simulink model "zynqRadioHWSWQPSKAD9361AD9364SL_orig"  (R2025a)
settings: Solver=FixedStepDiscrete  StartTime=0.0  StopTime=1e6/fs  RelTol=1e-3
PreLoadFcn:
  | setTxBurstLength = 10000;
  | txtmsg = ['Zynq radio HW/SW Co-design QPSK']; % Use only printable characters
  | 
  | %------------------------------------------------------------------------------------------------------
  | if ~isequal(size(txtmsg),[1 31])
  |     error('txtmsg must contain 31 characters');
  | end
  | 
  | [dataBits,msg] = zynqRadioHWSWQPSKgenHelloworldMsg(20); % generate 20 msgs for LUT
  | msgLUT = uint8(msg);
  | dataBitsLUT = dataBits(:);
  | Rsym                = 10e3;%1.92e6;
  | Config = zynqRadioHWSWQPSKTxRxParameters;
  | fs = Rsym*Config.SamplesPerSymbol;
  | word = [txtmsg newline];  % append a new line character to txtmsg
  | 
  | % The highest clock rate is 16 times the message character rate.
  | % As the message characters are fed at highest clock to FPGA
  | % repeat each character 16 times to maintain the message rate.
  | word = repelem(word.',16,1);
  | repeatTimes = ceil(setTxBurstLength/length(word));
  | inpData = complex(repmat(uint8(word),repeatTimes,1));
  | inUseTxBurstLength = length(inpData);
PostLoadFcn:
  | hScopeConfig = get_param([gcs '/HDL_QPSK/QPSK Tx Channel QPSK Rx/QPSK Rx/Frequency and Time Synchronizer/Symbol Synchronizer/No HDL/QPSK Receiver Eye Diagram'],'ScopeConfiguration');
  | hScopeConfig.OpenAtSimulationStart = false;
  | hScopeConfig.Visible = false;
  | clear hScopeConfig
InitFcn:
  | setTxBurstLength = 10000;
  | txtmsg = ['Zynq radio HW/SW Co-design QPSK']; % Use only printable characters
  | 
  | %------------------------------------------------------------------------------------------------------
  | if ~isequal(size(txtmsg),[1 31])
  |     error('txtmsg must contain 31 characters');
  | end
  | 
  | [dataBits,msg] = zynqRadioHWSWQPSKgenHelloworldMsg(20); % generate 20 msgs for LUT
  | msgLUT = uint8(msg);
  | dataBitsLUT = dataBits(:);
  | Rsym                = 10e3;%1.92e6;
  | Config = zynqRadioHWSWQPSKTxRxParameters;
  | fs = Rsym*Config.SamplesPerSymbol;
  | word = [txtmsg newline];  % append a new line character to txtmsg
  | 
  | % The highest clock rate is 16 times the message character rate.
  | % As the message characters are fed at highest clock to FPGA
  | % repeat each character 16 times to maintain the message rate.
  | word = repelem(word.',16,1);
  | repeatTimes = ceil(setTxBurstLength/length(word));
  | inpData = complex(repmat(uint8(word),repeatTimes,1));
  | inUseTxBurstLength = length(inpData);
undefined symbols (not defined in the file or in its folder): Add, DSP48_Variant, dspblkCoreblockFVToolHelper, gcbh, NCO_DUT, Shift, xc7z020clg484
libraries: hdlsllib x84, hdlBasic x50, simulink x34, dsphdlsigops2 x3, dsphdlfiltering2 x3, dsphdlxfrm2 x2, dsphdlmathfun2 x2, commdigbbndpm3 x2, vmcUtilities x1, sdrzblksprivate x1
(part 1 of 4)
CloseFcn:
  | clear Config dataBits dataBitsLUT fs h inpData ...
  |         inUseTxBurstLength msg msgLUT repeatTimes ...
  |         Rsym setTxBurstLength simAfterCS simBeforeSS ...
  |         simPeakFind simSyncedPackets simTimingOffset ...
  |         simUserData tout txtmsg word captureASCII
settings Model: DataTypeOverride=Off  Creator=The MathWorks, Inc.  LastModifiedBy=daniel
settings DataIOCC: ReturnWorkspaceOutputs=off
settings OptimizationCC: BlockReduction=off  ConditionallyExecuteInputs=off  DefaultParameterBehavior=Inlined  InheritOutputTypeSmallerThanSingle=on  ReuseModelBlockBuffer=off
settings DebuggingCC: AlgebraicLoopMsg=error  SingleTaskRateTransMsg=error  SubsystemReferenceDiagnosticForUnitTest=warning
settings HardwareCC: ProdBitPerPointer=32.0  ProdBitPerSizeT=32.0  ProdBitPerPtrDiffT=32.0  ProdLargestAtomicFloat=None  ProdIntDivRoundTo=Undefined  ProdEndianess=Unspecified  ProdWordSize=32.0  ProdHWDeviceType=ASIC/FPGA->ASIC/FPGA  TargetBitPerLong=64.0  TargetBitPerPointer=64.0  TargetBitPerSizeT=64.0  TargetBitPerPtrDiffT=64.0  TargetLongLongMode=on  TargetIntDivRoundTo=Zero  TargetEndianess=LittleEndian  TargetWordSize=64.0  TargetHWDeviceType=Custom Processor->MATLAB Host Computer  ProdEqTarget=off
settings RTWCC: GPUComputeCapability=3.5

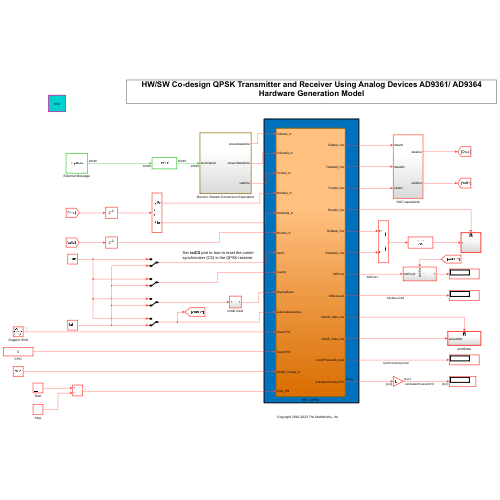
[thumbnail: Simulink's stored preview of the top-level diagram]
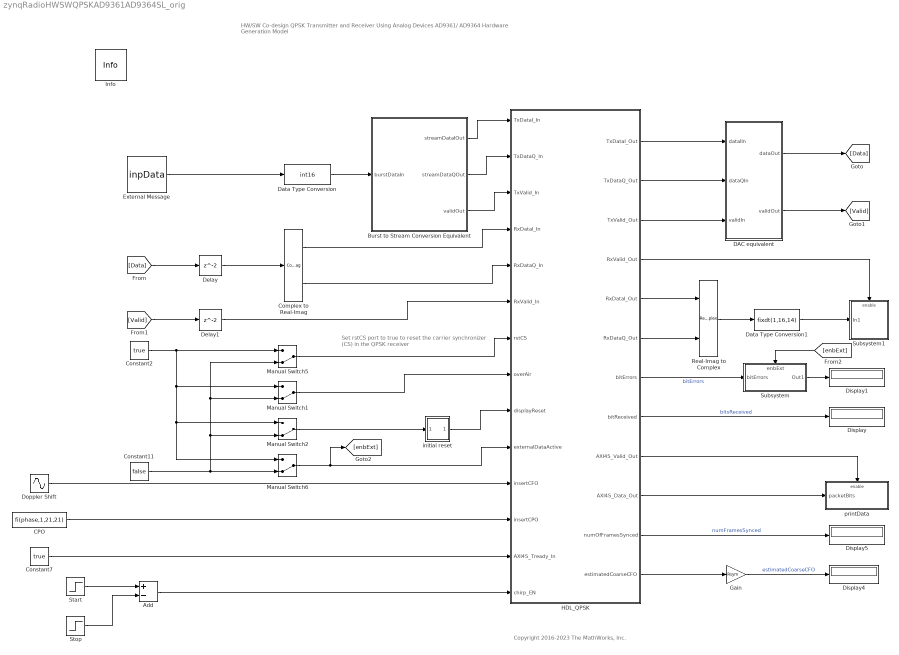
== system zynqRadioHWSWQPSKAD9361AD9364SL_orig ==
  note: Set rstCS port to true to reset the carrier synchronizer (CS) in the QPSK receiver
  note: Copyright 2016-2023 The MathWorks, Inc.
  note: HW/SW Co-design QPSK Transmitter and Receiver Using Analog Devices AD9361/ AD9364
      | Hardware Generation Model
  Add : Sum  Inputs=+-
  Burst to Stream Conversion Equivalent : Subsystem
  CPO : Constant  Value=fi(phase,1,21,21)  SampleTime=1/fs  mask{phased=0}
      mask prompts: phased "CPO (degrees):"
      mask init:
      | phase = phased/360;
      mask DialogControl DescGroupVar Prompt: Insert CPO
      mask DialogControl DescTextVar Prompt: Introduce CPO into transmitter waveform. The overAir port must be set to false. CPO range: -180 to less than 180
      mask Display: disp(get_param(gcb,"phased"));
  Complex to Real-Imag : ComplexToRealImag
  Constant11 : Constant  Value=false  OutDataTypeStr=boolean  SampleTime=1/fs
  Constant2 : Constant  Value=true  OutDataTypeStr=boolean  SampleTime=1/fs
  Constant7 : Constant  Value=true  OutDataTypeStr=boolean  SampleTime=1/fs
  DAC equivalent : Subsystem
  Data Type Conversion : DataTypeConversion  OutDataTypeStr=int16  SaturateOnIntegerOverflow=off  RndMeth=Floor
  Data Type Conversion1 : DataTypeConversion  OutDataTypeStr=fixdt(1,16,14)  ConvertRealWorld=Stored Integer (SI)  SaturateOnIntegerOverflow=off  RndMeth=Floor
  Delay : Delay
  Delay1 : Delay
  Display{,1,4..5} (4 alike) : Display
  Doppler Shift : Sin  SineType=Sample based  Amplitude=-100e3  Bias=100e3  Frequency=2*pi  Phase=pi  Samples=5*60*fs  SampleTime=1/fs
  External Message : Constant  Value=inpData  SampleTime=-1
  Gain : Gain  Gain=Rsym  OutDataTypeStr=double
  HDL_QPSK : Subsystem  TreatAsAtomicUnit=on
  Info : sdrzblksprivate/Info  SystemSampleTime=-1  VariantActivationTime=update diagram  EmptyChoice=off  PassThrough=off  PassThroughVariantControl=(default)  EmptyChoiceVariantControl=(default)  AllowFlexibleInterface=on  Latency=0  AutoFrameSizeCalculation=off
  Manual Switch{1..2,5..6} (4 alike) : ManualSwitch  CurrentSetting=0
  Real-Imag to Complex : RealImagToComplex
  Start : Step  Time=200e3/fs  SampleTime=1/fs
  Stop : Step  Time=400e3/fs  SampleTime=1/fs
  Subsystem : Subsystem
      settings: PortSchema="{\"entries\":[{\"content\":{\"sides\":[{\"content\":{\"connectorIds\":[\"In1\"]},\"type\":\"ConnectorPlacement.EquallySpacedRectSide\",\"uuid\":\"00e2ba4b-7eac-479c-adca-0b3a47f26300\"},{\"content\":{\"connectorIds\":[\"Out1\"],\"side\":\"RIGHT\"},\"type\":\"ConnectorPlacement.EquallySpacedRectSide\",\"uuid\":\"f46d1850-7aaf-4a4a-a0f0-18f53e4dd1ab\"},{\"content\":{\"connectorIds\":[\"In2\"],\"side\":\"TOP\"},\"type\":\"ConnectorPlacement.EquallySpacedRectSide\",\"uuid\":\"6eb79df9-d0ed-4616-8b56-bf03dd754f89\"}]},\"type\":\"ConnectorPlacement.EquallySpacedConnector\",\"uuid\":\"71623fc3-6fb3-42f9-b5c9-cd74da1aa0dd\"}],\"packageUris\":[\"http://schema.mathworks.com/mf0/Connector/R2020b\"],\"version\":\"1.0\"}"
  Subsystem1 : Subsystem
  initial reset : Subsystem
  printData : Subsystem
  wires:
  Doppler Shift/1 -> HDL_QPSK/11(insertCFO)
  Subsystem/1(Out1) -> Display1/1
  Complex to Real-Imag/1 -> HDL_QPSK/4(RxDataI_In)
  HDL_QPSK/1(TxDataI_Out) -> DAC equivalent/1(dataIIn)
  DAC equivalent/1(dataOut) -> [Data]
  [Valid] -> Delay1/1
  HDL_QPSK/2(TxDataQ_Out) -> DAC equivalent/2(dataQIn)
  HDL_QPSK/6(RxDataQ_Out) -> Real-Imag to Complex/2
  Manual Switch5/1 -> HDL_QPSK/7(rstCS)
  HDL_QPSK/12(estimatedCoarseCFO) -> Gain/1
  Delay1/1 -> HDL_QPSK/6(RxValid_In)
  CPO/1 -> HDL_QPSK/12(insertCPO)
  Manual Switch1/1 -> HDL_QPSK/8(overAir)
  HDL_QPSK/9(AXI4S_Valid_Out) -> printData/Enable
  Real-Imag to Complex/1 -> Data Type Conversion1/1
  Data Type Conversion1/1 -> Subsystem1/1(In1)
  HDL_QPSK/4(RxValid_Out) -> Subsystem1/Enable
  HDL_QPSK/10(AXI4S_Data_Out) -> printData/1(packetBits)
  External Message/1 -> Data Type Conversion/1
  Constant7/1 -> HDL_QPSK/13(AXI4S_Tready_In)
  Burst to Stream Conversion Equivalent/3(validOut) -> HDL_QPSK/3(TxValid_In)
  DAC equivalent/2(validOut) -> [Valid]
  Burst to Stream Conversion Equivalent/1(streamDataIOut) -> HDL_QPSK/1(TxDataI_In)
  Gain/1 -> Display4/1  "estimatedCoarseCFO"
  Delay/1 -> Complex to Real-Imag/1
  HDL_QPSK/7(bitErrors) -> Subsystem/1(bitErrors)  "bitErrors"
  HDL_QPSK/11(numOfFramesSynced) -> Display5/1  "numFramesSynced"
  HDL_QPSK/3(TxValid_Out) -> DAC equivalent/3(validIn)
  [enbExt] -> Subsystem/2(enbExt)
  Manual Switch2/1 -> initial reset/1(In2)
  initial reset/1(Out1) -> HDL_QPSK/9(displayReset)
  Constant2/1 -> Manual Switch6/1, Manual Switch2/1, Manual Switch1/1, Manual Switch5/1
  Burst to Stream Conversion Equivalent/2(streamDataQOut) -> HDL_QPSK/2(TxDataQ_In)
  Constant11/1 -> Manual Switch6/2, Manual Switch5/2, Manual Switch1/2, Manual Switch2/2
  HDL_QPSK/5(RxDataI_Out) -> Real-Imag to Complex/1
  Data Type Conversion/1 -> Burst to Stream Conversion Equivalent/1(burstDataIn)
  Complex to Real-Imag/2 -> HDL_QPSK/5(RxDataQ_In)
  HDL_QPSK/8(bitReceived) -> Display/1  "bitsReceived"
  [Data] -> Delay/1
  Manual Switch6/1 -> HDL_QPSK/10(externalDataActive), [enbExt]
  Start/1 -> Add/1
  Stop/1 -> Add/2
  Add/1 -> HDL_QPSK/14(chirp_EN)

== system zynqRadioHWSWQPSKAD9361AD9364SL_orig/Burst to Stream Conversion Equivalent ==
  note: The burst data sent from the processing system will be stored in the RAM in the memory channel of SDR IIO radio. The data stored will be poped out as a stream data.
  note: This subsystem does an equivalent operation to simulate the input and output behaviour of the memory channel of the SDR IIO radio.
  burstDataIn : Inport
  Complex to Real-Imag : ComplexToRealImag
  Serializer1D : hdlsllib/HDL Operations/Serializer1D  Ratio=inUseTxBurstLength  IdleCycles=0  validIn=off  startOut=off  validOut=on  inputDataDimensions=-1  inputSampleTime=-1  inputSignalType=auto
  streamDataIOut : Outport
  streamDataQOut : Outport  Port=2
  validOut : Outport  Port=3
  wires:
  burstDataIn/1 -> Serializer1D/1
  Serializer1D/1 -> Complex to Real-Imag/1
  Complex to Real-Imag/1 -> streamDataIOut/1
  Complex to Real-Imag/2 -> streamDataQOut/1
  Serializer1D/2 -> validOut/1

== system zynqRadioHWSWQPSKAD9361AD9364SL_orig/DAC equivalent ==
  dataIIn : Inport
  dataQIn : Inport  Port=2
  validIn : Inport  Port=3
  Data Type Conversion : DataTypeConversion  OutDataTypeStr=int16  SaturateOnIntegerOverflow=off  RndMeth=Floor
  Extract Bits : simulink/Logic and Bit Operations/Extract Bits  bitsToExtract=Range starting with most significant bit  numBits=12  bitIdxRange=[0 7]  outScalingMode=Treat bit field as an integer
  Extract Bits1 : simulink/Logic and Bit Operations/Extract Bits  bitsToExtract=Range starting with most significant bit  numBits=12  bitIdxRange=[0 7]  outScalingMode=Treat bit field as an integer
  Real-Imag to Complex : RealImagToComplex
  dataOut : Outport
  validOut : Outport  Port=2
  wires:
  dataIIn/1 -> Extract Bits/1
  dataQIn/1 -> Extract Bits1/1
  Extract Bits/1 -> Real-Imag to Complex/1
  Extract Bits1/1 -> Real-Imag to Complex/2
  Real-Imag to Complex/1 -> Data Type Conversion/1
  validIn/1 -> validOut/1
  Data Type Conversion/1 -> dataOut/1

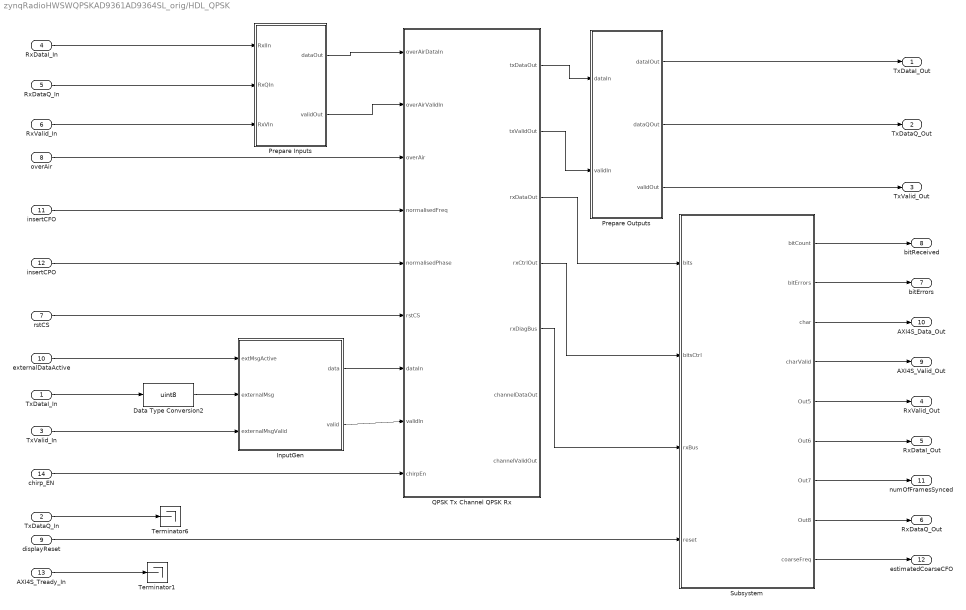
== system zynqRadioHWSWQPSKAD9361AD9364SL_orig/HDL_QPSK ==
  TxDataI_In : Inport
  TxDataQ_In : Inport  Port=2
  TxValid_In : Inport  Port=3
  RxDataI_In : Inport  Port=4
  RxDataQ_In : Inport  Port=5
  RxValid_In : Inport  Port=6
  rstCS : Inport  Port=7
  overAir : Inport  Port=8
  displayReset : Inport  Port=9
  externalDataActive : Inport  Port=10
  insertCFO : Inport  Port=11
  insertCPO : Inport  Port=12
  AXI4S_Tready_In : Inport  Port=13
  chirp_EN : Inport  Port=14
  Data Type Conversion2 : DataTypeConversion  OutDataTypeStr=uint8  SaturateOnIntegerOverflow=off  RndMeth=Floor
  InputGen : Subsystem
  Prepare Inputs : Subsystem
  Prepare Outputs : Subsystem
  QPSK Tx Channel QPSK Rx : Subsystem
  Subsystem : Subsystem
  Terminator1 : Terminator
  Terminator6 : Terminator
  TxDataI_Out : Outport
  TxDataQ_Out : Outport  Port=2
  TxValid_Out : Outport  Port=3
  RxValid_Out : Outport  Port=4
  RxDataI_Out : Outport  Port=5
  RxDataQ_Out : Outport  Port=6
  bitErrors : Outport  Port=7
  bitReceived : Outport  Port=8
  AXI4S_Valid_Out : Outport  Port=9
  AXI4S_Data_Out : Outport  Port=10
  numOfFramesSynced : Outport  Port=11
  estimatedCoarseCFO : Outport  Port=12
  wires:
  Prepare Outputs/2(dataQOut) -> TxDataQ_Out/1
  Prepare Outputs/3(validOut) -> TxValid_Out/1
  AXI4S_Tready_In/1 -> Terminator1/1
  Prepare Inputs/1(dataOut) -> QPSK Tx Channel QPSK Rx/1(overAirDataIn)
  Prepare Inputs/2(validOut) -> QPSK Tx Channel QPSK Rx/2(overAirValidIn)
  InputGen/1(data) -> QPSK Tx Channel QPSK Rx/7(dataIn)
  InputGen/2(valid) -> QPSK Tx Channel QPSK Rx/8(validIn)
  overAir/1 -> QPSK Tx Channel QPSK Rx/3(overAir)
  insertCFO/1 -> QPSK Tx Channel QPSK Rx/4(normalisedFreq)
  insertCPO/1 -> QPSK Tx Channel QPSK Rx/5(normalisedPhase)
  QPSK Tx Channel QPSK Rx/1(txDataOut) -> Prepare Outputs/1(dataIn)
  QPSK Tx Channel QPSK Rx/2(txValidOut) -> Prepare Outputs/2(validIn)
  displayReset/1 -> Subsystem/4(reset)
  QPSK Tx Channel QPSK Rx/3(rxDataOut) -> Subsystem/1(bits)
  QPSK Tx Channel QPSK Rx/4(rxCtrlOut) -> Subsystem/2(bitsCtrl)
  QPSK Tx Channel QPSK Rx/5(rxDiagBus) -> Subsystem/3(rxBus)
  Subsystem/1(bitCount) -> bitReceived/1
  Subsystem/2(bitErrors) -> bitErrors/1
  Subsystem/3(char) -> AXI4S_Data_Out/1
  Subsystem/4(charValid) -> AXI4S_Valid_Out/1
  Subsystem/5(Out5) -> RxValid_Out/1
  Subsystem/6(Out6) -> RxDataI_Out/1
  Subsystem/7(Out7) -> numOfFramesSynced/1
  Subsystem/8(Out8) -> RxDataQ_Out/1
  rstCS/1 -> QPSK Tx Channel QPSK Rx/6(rstCS)
  Subsystem/9(coarseFreq) -> estimatedCoarseCFO/1
  Prepare Outputs/1(dataIOut) -> TxDataI_Out/1
  RxDataI_In/1 -> Prepare Inputs/1(RxIIn)
  RxDataQ_In/1 -> Prepare Inputs/2(RxQIn)
  RxValid_In/1 -> Prepare Inputs/3(RxVIn)
  TxValid_In/1 -> InputGen/3(externalMsgValid)
  TxDataQ_In/1 -> Terminator6/1
  externalDataActive/1 -> InputGen/1(extMsgActive)
  TxDataI_In/1 -> Data Type Conversion2/1
  Data Type Conversion2/1 -> InputGen/2(externalMsg)
  chirp_EN/1 -> QPSK Tx Channel QPSK Rx/9(chirpEn)

== system zynqRadioHWSWQPSKAD9361AD9364SL_orig/Subsystem ==
  note: 2^32-1 will be treated as NaN in double when converted to double
  bitErrors : Inport
  enbExt : Inport  Port=2
  Compare To Constant : simulink/Logic and Bit Operations/Compare To Constant  relop===  const=2^32-1  OutDataTypeStr=boolean
  Constant : Constant  Value=2^32-1  OutDataTypeStr=uint32  SampleTime=-1
  Constant1 : Constant  Value=NaN  SampleTime=-1
  Data Type Conversion3 : DataTypeConversion  OutDataTypeStr=double  SaturateOnIntegerOverflow=off  RndMeth=Floor
  Switch : Switch  Criteria=u2 ~= 0  SaturateOnIntegerOverflow=off  InputSameDT=off
  Switch1 : Switch  Criteria=u2 ~= 0  SaturateOnIntegerOverflow=off  InputSameDT=off
  Out1 : Outport
  wires:
  Constant/1 -> Switch/1
  bitErrors/1 -> Switch/3
  enbExt/1 -> Switch/2
  Compare To Constant/1 -> Switch1/2
  Switch1/1 -> Out1/1
  Switch/1 -> Data Type Conversion3/1, Compare To Constant/1
  Data Type Conversion3/1 -> Switch1/3
  Constant1/1 -> Switch1/1

== system zynqRadioHWSWQPSKAD9361AD9364SL_orig/Subsystem1 ==
  In1 : Inport
  Enable : EnablePort
  Constellation Diagram : ConstellationDiagram  WindowPosition=[499.000000,206.000000,1692.000000,1017.000000,]  ScopeFrameLocation=window  SymbolsToDisplaySource=Property  SymbolsToDisplay=10000  XLimits=[-1.38,1.38]  YLimits=[-1.38,1.38]  AxesLimits=[-1.38,1.38]  DefaultConfigurationName=comm.scopes.ConstellationDiagramBlockCfg
  Terminator : Terminator
  wires:
  In1/1 -> Constellation Diagram/1, Terminator/1

== system zynqRadioHWSWQPSKAD9361AD9364SL_orig/initial reset ==
  In2 : Inport
  Constant : Constant  OutDataTypeStr=boolean  SampleTime=-1
  Delay : Delay  DelayLength=1
  Logical Operator : Logic  Operator=OR  IconShape=distinctive  AllPortsSameDT=off  OutDataTypeStr=boolean
  Logical Operator1 : Logic  Operator=XOR  IconShape=distinctive  AllPortsSameDT=off  OutDataTypeStr=boolean
  Out1 : Outport
  wires:
  In2/1 -> Logical Operator/2
  Logical Operator1/1 -> Logical Operator/1
  Logical Operator/1 -> Out1/1
  Constant/1 -> Delay/1, Logical Operator1/1
  Delay/1 -> Logical Operator1/2

== system zynqRadioHWSWQPSKAD9361AD9364SL_orig/printData ==
  packetBits : Inport
  Enable : EnablePort
  Extract Bits : simulink/Logic and Bit Operations/Extract Bits  bitsToExtract=Range ending with least significant bit  numBits=8  bitIdxRange=[0 7]  outScalingMode=Treat bit field as an integer
  MATLAB Function : MATLAB Function  TreatAsAtomicUnit=on
  Serializer1D : hdlsllib/HDL Operations/Serializer1D  Ratio=1  IdleCycles=0  validIn=off  startOut=off  validOut=off  inputDataDimensions=-1  inputSampleTime=-1  inputSignalType=auto
  captureASCII : ToWorkspace  VariableName=captureASCII  SampleTime=-1
      settings: Save2DSignal=2-D array (concatenate along first dimension)
  wires:
  packetBits/1 -> Serializer1D/1
  Serializer1D/1 -> Extract Bits/1
  Extract Bits/1 -> captureASCII/1, MATLAB Function/1(u)

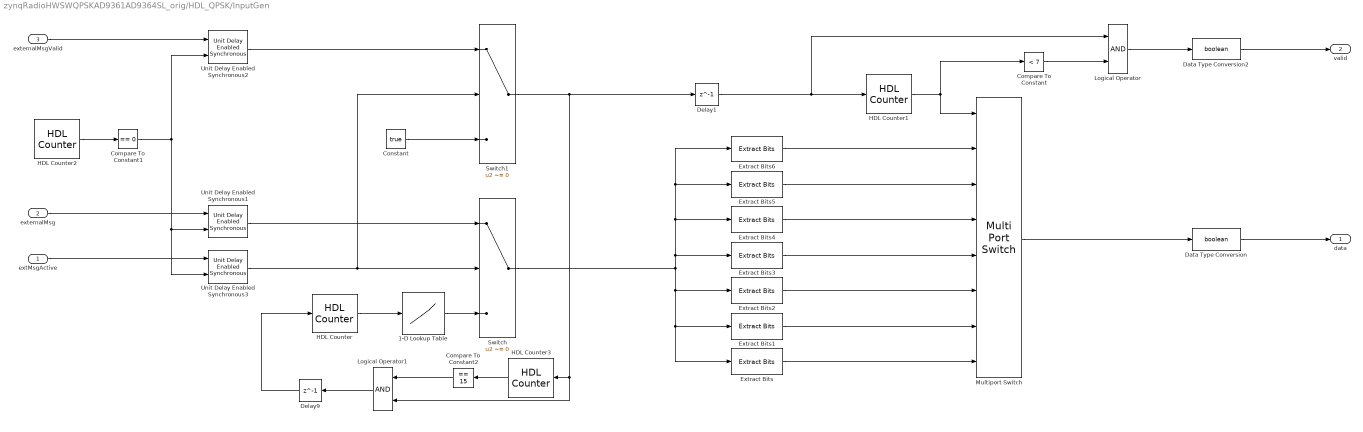
== system zynqRadioHWSWQPSKAD9361AD9364SL_orig/HDL_QPSK/InputGen ==
  extMsgActive : Inport
  externalMsg : Inport  Port=2
  externalMsgValid : Inport  Port=3
  1-D Lookup Table : Lookup_n-D  NumberOfTableDimensions=1  LookupTableObject=''  BreakpointsForDimension1=0:length(msgLUT) - 1  BreakpointsForDimension1FirstPoint=10  BreakpointsForDimension2FirstPoint=10  BreakpointsForDimension1Spacing=12  BreakpointsForDimension2Spacing=12  IndexSearchMethod=Evenly spaced points  Table=msgLUT  TableDataTypeStr=uint8  InterpMethod=Flat  DiagnosticForOutOfRangeInput=Error  InternalRulePriority=Speed  OutDataTypeStr=uint8  RndMeth=Simplest
  Compare To Constant : simulink/Logic and Bit Operations/Compare To Constant  relop=<  const=7  OutDataTypeStr=boolean
  Compare To Constant1 : hdlsllib/Logic and Bit Operations/Compare To Constant  relop===  const=0  OutDataTypeStr=boolean
  Compare To Constant2 : hdlsllib/Logic and Bit Operations/Compare To Constant  relop===  const=15  OutDataTypeStr=boolean
  Constant : Constant  Value=true  SampleTime=-1
  Data Type Conversion : DataTypeConversion  OutDataTypeStr=boolean  SaturateOnIntegerOverflow=off  RndMeth=Floor
  Data Type Conversion2 : DataTypeConversion  OutDataTypeStr=boolean  SaturateOnIntegerOverflow=off  RndMeth=Floor
  Delay1 : Delay  DelayLength=1
  Delay9 : Delay  DelayLength=1
  Extract Bits : simulink/Logic and Bit Operations/Extract Bits  bitsToExtract=Range of bits  numBits=8  bitIdxRange=0  outScalingMode=Treat bit field as an integer
  Extract Bits1 : simulink/Logic and Bit Operations/Extract Bits  bitsToExtract=Range of bits  numBits=8  bitIdxRange=1  outScalingMode=Treat bit field as an integer
  Extract Bits2 : simulink/Logic and Bit Operations/Extract Bits  bitsToExtract=Range of bits  numBits=8  bitIdxRange=2  outScalingMode=Treat bit field as an integer
  Extract Bits3 : simulink/Logic and Bit Operations/Extract Bits  bitsToExtract=Range of bits  numBits=8  bitIdxRange=3  outScalingMode=Treat bit field as an integer
  Extract Bits4 : simulink/Logic and Bit Operations/Extract Bits  bitsToExtract=Range of bits  numBits=8  bitIdxRange=4  outScalingMode=Treat bit field as an integer
  Extract Bits5 : simulink/Logic and Bit Operations/Extract Bits  bitsToExtract=Range of bits  numBits=8  bitIdxRange=5  outScalingMode=Treat bit field as an integer
  Extract Bits6 : simulink/Logic and Bit Operations/Extract Bits  bitsToExtract=Range of bits  numBits=8  bitIdxRange=6  outScalingMode=Treat bit field as an integer
  HDL Counter : hdlsllib/Sources/HDL Counter  CountType=Count limited  CountInit=0  CountStep=1  CountMax=length(msgLUT) - 1  CountFromType=Initial value  CountFrom=0  CountResetPort=off  CountLoadPort=off  CountEnbPort=on  CountDirPort=off  CountHitOutputPort=off  CountDataType=Unsigned  CountWordLen=nextpow2(length(msgLUT) - 1)  CountFracLen=0  CountSampTime=8/(Rsym*2)
  HDL Counter1 : hdlsllib/Sources/HDL Counter  CountType=Count limited  CountInit=0  CountStep=1  CountMax=15  CountFromType=Initial value  CountFrom=0  CountResetPort=off  CountLoadPort=off  CountEnbPort=on  CountDirPort=off  CountHitOutputPort=off  CountDataType=Unsigned  CountWordLen=4  CountFracLen=0  CountSampTime=1
  HDL Counter2 : hdlsllib/Sources/HDL Counter  CountType=Count limited  CountInit=0  CountStep=1  CountMax=15  CountFromType=Initial value  CountFrom=0  CountResetPort=off  CountLoadPort=off  CountEnbPort=off  CountDirPort=off  CountHitOutputPort=off  CountDataType=Unsigned  CountWordLen=4  CountFracLen=0  CountSampTime=1/fs
  HDL Counter3 : hdlsllib/Sources/HDL Counter  CountType=Count limited  CountInit=0  CountStep=1  CountMax=15  CountFromType=Initial value  CountFrom=0  CountResetPort=off  CountLoadPort=off  CountEnbPort=on  CountDirPort=off  CountHitOutputPort=off  CountDataType=Unsigned  CountWordLen=4  CountFracLen=0  CountSampTime=1/fs
  Logical Operator : Logic  AllPortsSameDT=off  OutDataTypeStr=boolean
  Logical Operator1 : Logic  AllPortsSameDT=off  OutDataTypeStr=boolean
  Multiport Switch : MultiPortSwitch  DataPortOrder=Zero-based contiguous  Inputs=7  DiagnosticForDefault=None  zeroidx=on  SaturateOnIntegerOverflow=off  InputSameDT=off
  Switch : Switch  Criteria=u2 ~= 0  SaturateOnIntegerOverflow=off  InputSameDT=off
  Switch1 : Switch  Criteria=u2 ~= 0  SaturateOnIntegerOverflow=off  InputSameDT=off
  Unit Delay Enabled Synchronous1 : hdlsllib/Discrete/Unit Delay Enabled Synchronous  InitialCondition=0.0  SampleTime=-1
  Unit Delay Enabled Synchronous2 : hdlsllib/Discrete/Unit Delay Enabled Synchronous  InitialCondition=0.0  SampleTime=-1
  Unit Delay Enabled Synchronous3 : hdlsllib/Discrete/Unit Delay Enabled Synchronous  InitialCondition=0.0  SampleTime=-1
  data : Outport
  valid : Outport  Port=2
  wires:
  Logical Operator1/1 -> Delay9/1
  Compare To Constant2/1 -> Logical Operator1/1
  HDL Counter3/1 -> Compare To Constant2/1
  Delay1/1 -> Logical Operator/1, HDL Counter1/1
  Constant/1 -> Switch1/3
  Extract Bits/1 -> Multiport Switch/8
  Extract Bits1/1 -> Multiport Switch/7
  Extract Bits2/1 -> Multiport Switch/6
  Extract Bits3/1 -> Multiport Switch/5
  Extract Bits4/1 -> Multiport Switch/4
  Extract Bits5/1 -> Multiport Switch/3
  Extract Bits6/1 -> Multiport Switch/2
  Unit Delay Enabled Synchronous3/1 -> Switch/2, Switch1/2
  extMsgActive/1 -> Unit Delay Enabled Synchronous3/1
  Unit Delay Enabled Synchronous2/1 -> Switch1/1
  externalMsg/1 -> Unit Delay Enabled Synchronous1/1
  Compare To Constant1/1 -> Unit Delay Enabled Synchronous1/2, Unit Delay Enabled Synchronous3/2, Unit Delay Enabled Synchronous2/2
  externalMsgValid/1 -> Unit Delay Enabled Synchronous2/1
  HDL Counter2/1 -> Compare To Constant1/1
  Unit Delay Enabled Synchronous1/1 -> Switch/1
  Delay9/1 -> HDL Counter/1
  Switch/1 -> Extract Bits3/1, Extract Bits4/1, Extract Bits5/1, Extract Bits6/1, Extract Bits2/1, Extract Bits1/1, Extract Bits/1
  Logical Operator/1 -> Data Type Conversion2/1
  Switch1/1 -> Delay1/1, HDL Counter3/1, Logical Operator1/2
  1-D Lookup Table/1 -> Switch/3
  Compare To Constant/1 -> Logical Operator/2
  HDL Counter1/1 -> Multiport Switch/1, Compare To Constant/1
  Multiport Switch/1 -> Data Type Conversion/1
  HDL Counter/1 -> 1-D Lookup Table/1
  Data Type Conversion/1 -> data/1
  Data Type Conversion2/1 -> valid/1

== system zynqRadioHWSWQPSKAD9361AD9364SL_orig/HDL_QPSK/Prepare Inputs ==
  RxIIn : Inport
  RxQIn : Inport  Port=2
  RxVIn : Inport  Port=3
  Data Type Conversion5 : DataTypeConversion  OutDataTypeStr=fixdt(1,16,14)  ConvertRealWorld=Stored Integer (SI)  SaturateOnIntegerOverflow=off  RndMeth=Floor
  Delay{1,3..4,6} (4 alike) : Delay
  Delay2 : Delay  DelayLength=4
  Delay5 : Delay  DelayLength=4
  Gain : Gain  Gain=16  ParamDataTypeStr=fixdt(0,5,0)  OutDataTypeStr=Inherit: Same as input
  Real-Imag to Complex : RealImagToComplex
  dataOut : Outport
  validOut : Outport  Port=2
  wires:
  RxIIn/1 -> Real-Imag to Complex/1
  Gain/1 -> Delay2/1
  Real-Imag to Complex/1 -> Data Type Conversion5/1
  Delay5/1 -> Delay6/1
  Data Type Conversion5/1 -> Delay1/1
  Delay2/1 -> Delay3/1
  Delay4/1 -> Delay5/1
  RxQIn/1 -> Real-Imag to Complex/2
  Delay1/1 -> Gain/1
  RxVIn/1 -> Delay4/1
  Delay6/1 -> validOut/1
  Delay3/1 -> dataOut/1

== system zynqRadioHWSWQPSKAD9361AD9364SL_orig/HDL_QPSK/Prepare Outputs ==
  dataIn : Inport
  validIn : Inport  Port=2
  Complex to Real-Imag1 : ComplexToRealImag
  Data Type Conversion4 : DataTypeConversion  OutDataTypeStr=int16  ConvertRealWorld=Stored Integer (SI)  SaturateOnIntegerOverflow=off  RndMeth=Floor
  Delay7 : Delay
  Delay8 : Delay
  Delay9 : Delay
  dataIOut : Outport
  dataQOut : Outport  Port=2
  validOut : Outport  Port=3
  wires:
  dataIn/1 -> Data Type Conversion4/1
  Delay7/1 -> dataIOut/1
  Complex to Real-Imag1/2 -> Delay8/1
  validIn/1 -> Delay9/1
  Complex to Real-Imag1/1 -> Delay7/1
  Data Type Conversion4/1 -> Complex to Real-Imag1/1
  Delay9/1 -> validOut/1
  Delay8/1 -> dataQOut/1

== system zynqRadioHWSWQPSKAD9361AD9364SL_orig/HDL_QPSK/QPSK Tx Channel QPSK Rx ==
  overAirDataIn : Inport
  overAirValidIn : Inport  Port=2
  overAir : Inport  Port=3
  normalisedFreq : Inport  Port=4
  normalisedPhase : Inport  Port=5
  rstCS : Inport  Port=6
  dataIn : Inport  Port=7
  validIn : Inport  Port=8
  chirpEn : Inport  Port=9
  Data Type Conversion7 : DataTypeConversion  OutDataTypeStr=fixdt(1,16,14)  SaturateOnIntegerOverflow=off  RndMeth=Floor
  QPSK Rx : Subsystem
      mask init:
      | integAvgLen = 2^15;
      | 
      | RxParams            = zynqRadioHWSWQPSKTxRxParameters();
      | Preamble            = RxParams.Preamble;
      | QPSKConstellation   = RxParams.QPSKConstellation;
      | dataBitsPerPacket   = RxParams.DataBitsPerPacket;
      | SamplesPerSymbol    = RxParams.SamplesPerSymbol;
      | RRCCoef             = RxParams.RRCCoef;
      | bitsPerPacket        = RxParams.BitsPerPacket;
      | 
      | rxPreambleMFCoeffs  = RxParams.rxPreambleMFCoeffs;
      | preambleSymbols     = RxParams.preambleSymbols;
      | ThresoldGainFac     = RxParams.ThresoldGainFac;
      | 
      | % AGC Parameters
      | AGCReference           = RxParams.AGCReference;
      | AGCLoopGain            = RxParams.AGCLoopGain;
      | 
      | % CS parameters
      | CSKp                   = RxParams.CSKp;
      | CSK0                   = RxParams.CSK0;  
      | CSLoopFilterPropGain   = RxParams.CSLoopFilterPropGain;
      | CSLoopFilterIntegGain  = RxParams.CSLoopFilterIntegGain;
      | CFOChangeDetectThreshold = RxParams.CFOChangeDetectThreshold;
      | 
      | % SS parameters
      | SSKp                   = RxParams.SSKp; 
      | SSK0                   = RxParams.SSK0;  
      | SSLoopFilterPropGain   = RxParams.SSLoopFilterPropGain;
      | SSLoopFilterIntegGain  = RxParams.SSLoopFilterIntegGain;
      | 
      | % preamble detector parameters
      | searchSamples          = RxParams.SearchSamples;
      | 
      | clear RxParams;
  QPSK Tx : Subsystem
      mask init:
      | TxParams            = zynqRadioHWSWQPSKTxRxParameters();
      | Preamble            = TxParams.Preamble;
      | QPSKConstellation   = TxParams.QPSKConstellation;
      | dataBitsPerPacket   = TxParams.DataBitsPerPacket;
      | SamplesPerSymbol    = TxParams.SamplesPerSymbol;
      | RRCCoef             = TxParams.RRCCoef;
      | dataRAMAddrWidth    = TxParams.txDataRAMAddrWidth;
      | bitsPerPacket       = TxParams.BitsPerPacket;
      | 
      | clear TxParams;
  Switch : Switch  Criteria=u2 ~= 0  Threshold=1  SaturateOnIntegerOverflow=off  InputSameDT=off
  Switch3 : Switch  Criteria=u2 ~= 0  Threshold=1  SaturateOnIntegerOverflow=off  InputSameDT=off
  Terminator : Terminator
  Terminator1 : Terminator
  channel : Subsystem
  txDataOut : Outport
  txValidOut : Outport  Port=2
  rxDataOut : Outport  Port=3
  rxCtrlOut : Outport  Port=4
  rxDiagBus : Outport  Port=5
  channelDataOut : Outport  Port=6
  channelValidOut : Outport  Port=7
  wires:
  dataIn/1 -> QPSK Tx/1(dataIn)
  QPSK Rx/3(rxDiagBus) -> rxDiagBus/1
  QPSK Tx/3(txDiagBus) -> Terminator1/1
  QPSK Rx/1(dataOut) -> rxDataOut/1
  QPSK Rx/2(ctrlOut) -> rxCtrlOut/1
  Data Type Conversion7/1 -> QPSK Rx/1(dataIn)
  Switch3/1 -> QPSK Rx/2(validIn)
  validIn/1 -> QPSK Tx/2(validIn)
  Switch/1 -> Data Type Conversion7/1
  normalisedPhase/1 -> channel/4(normalisedPhase)
  normalisedFreq/1 -> channel/3(normalisedFreq)
  QPSK Tx/4(validOut) -> channel/2(validIn), txValidOut/1
  QPSK Tx/2(dataOut) -> txDataOut/1, channel/1(dataIn)
  overAir/1 -> Switch3/2, Switch/2
  rstCS/1 -> QPSK Rx/3(rstCS)
  overAirDataIn/1 -> Switch/1
  overAirValidIn/1 -> Switch3/1
  channel/2(validOut) -> channelValidOut/1, Switch3/3
  channel/1(dataOut) -> channelDataOut/1, Switch/3
  QPSK Tx/1(dataReady) -> Terminator/1
  chirpEn/1 -> channel/5(chirpEn)

== system zynqRadioHWSWQPSKAD9361AD9364SL_orig/HDL_QPSK/Subsystem ==
  bits : Inport
  bitsCtrl : Inport  Port=2
  rxBus : Inport  Port=3
  reset : Inport  Port=4
  BER : Subsystem
  Bits to Char : Subsystem
  Bus Selector1 : BusSelector  OutputSignals=startOut,validOut
  Bus Selector2 : BusSelector  OutputSignals=nSynced,QPSKConstellationValid,QPSKConstellationPoints,normCoarseFreqEst
  Complex to Real-Imag : ComplexToRealImag
  Data Type Conversion1 : DataTypeConversion  OutDataTypeStr=int16  ConvertRealWorld=Stored Integer (SI)  SaturateOnIntegerOverflow=off  RndMeth=Floor
  Data Type Conversion3 : DataTypeConversion  OutDataTypeStr=uint32  SaturateOnIntegerOverflow=off  RndMeth=Floor
  HDL Counter : hdlsllib/Sources/HDL Counter  CountType=Free running  CountInit=0  CountStep=1  CountMax=25  CountFromType=Initial value  CountFrom=0  CountResetPort=on  CountLoadPort=off  CountEnbPort=on  CountDirPort=off  CountHitOutputPort=off  CountDataType=Unsigned  CountWordLen=32  CountFracLen=0  CountSampTime=1
  bitCount : Outport
  bitErrors : Outport  Port=2
  char : Outport  Port=3
  charValid : Outport  Port=4
  Out5 : Outport  Port=5
  Out6 : Outport  Port=6
  Out7 : Outport  Port=7
  Out8 : Outport  Port=8
  coarseFreq : Outport  Port=9
  wires:
  rxBus/1 -> Bus Selector2/1
  Data Type Conversion3/1 -> char/1
  Complex to Real-Imag/2 -> Out8/1
  HDL Counter/1 -> Out7/1
  Complex to Real-Imag/1 -> Out6/1
  BER/2(bitErrors) -> bitErrors/1
  Bits to Char/2(charValid) -> charValid/1
  BER/1(bitCount) -> bitCount/1
  Data Type Conversion1/1 -> Complex to Real-Imag/1
  Bus Selector2/2 -> Out5/1  "<QPSKConstellationValid>"
  Bus Selector2/1 -> HDL Counter/2  "<nSynced>"
  bits/1 -> Bits to Char/1(data), BER/4(userBits)
  Bits to Char/1(charOut) -> Data Type Conversion3/1
  bitsCtrl/1 -> Bus Selector1/1
  Bus Selector2/3 -> Data Type Conversion1/1  "<QPSKConstellationPoints>"
  Bus Selector1/2 -> BER/1(userBitsValid), Bits to Char/3(valid)  "<validOut>"
  Bus Selector1/1 -> BER/2(resetcounter), Bits to Char/2(start)  "<startOut>"
  Bus Selector2/4 -> coarseFreq/1  "<normCoarseFreqEst>"
  reset/1 -> HDL Counter/1, BER/3(reset)

== system zynqRadioHWSWQPSKAD9361AD9364SL_orig/HDL_QPSK/QPSK Tx Channel QPSK Rx/QPSK Rx ==
  dataIn : Inport  OutDataTypeStr=fixdt(1,16,14)  PortDimensions=1  SampleTime=1/(Rsym*SamplesPerSymbol)
      settings: SignalType=complex
  validIn : Inport  Port=2  OutDataTypeStr=boolean  PortDimensions=1  SampleTime=1/(Rsym*SamplesPerSymbol)
  rstCS : Inport  Port=3  OutDataTypeStr=boolean  PortDimensions=1
      settings: SignalType=complex
  Automatic Gain Control : Subsystem  mask{Ref=AGCReference, LFG=AGCLoopGain}
      mask prompts: Ref "Error Detector Reference:"; LFG "Loop Filter Gain"
  Bus Creator : BusCreator  Inputs=4
  Bus Creator1 : BusCreator  Inputs=3
  Delay : Delay  DelayLength=1
  FRFT Interference Cancellation : Subsystem  Commented=on
      settings: PortSchema="{\"entries\":[{\"content\":{\"sides\":[{\"content\":{\"connectorIds\":[\"In1\",\"In2\"]},\"type\":\"ConnectorPlacement.EquallySpacedRectSide\",\"uuid\":\"50491e4b-448d-4897-93d5-82658af40e6a\"},{\"content\":{\"connectorIds\":[\"Out1\",\"Out2\"],\"side\":\"RIGHT\"},\"type\":\"ConnectorPlacement.EquallySpacedRectSide\",\"uuid\":\"92b7170a-fe32-477b-a0aa-07b62d03a88a\"},{\"content\":{\"connectorIds\":[\"In3\"],\"side\":\"TOP\"},\"type\":\"ConnectorPlacement.EquallySpacedRectSide\",\"uuid\":\"ae8eeabd-9a0c-434e-a24f-48ab553d0b87\"}]},\"type\":\"ConnectorPlacement.EquallySpacedConnector\",\"uuid\":\"9bc37ce9-ba4c-4d42-a736-75d3eb39cc46\"}],\"packageUris\":[\"http://schema.mathworks.com/mf0/Connector/R2020b\"],\"version\":\"1.0\"}"
  Frequency and Time Synchronizer : Subsystem
      settings: PortSchema="{\"entries\":[{\"content\":{\"sides\":[{\"content\":{\"connectorIds\":[\"In1\",\"In2\"]},\"type\":\"ConnectorPlacement.EquallySpacedRectSide\",\"uuid\":\"8bc6a452-5111-4806-8ca9-335cb622aea6\"},{\"content\":{\"connectorIds\":[\"Out1\",\"Out2\",\"Out3\",\"Out4\"],\"side\":\"RIGHT\"},\"type\":\"ConnectorPlacement.EquallySpacedRectSide\",\"uuid\":\"b0f43c98-f5c0-4f62-94ae-d69789942eef\"},{\"content\":{\"connectorIds\":[\"In3\",\"Out5\",\"Out6\"],\"side\":\"TOP\"},\"type\":\"ConnectorPlacement.EquallySpacedRectSide\",\"uuid\":\"427ff3b3-b896-4008-9584-d311480df763\"},{\"content\":{\"connectorIds\":[],\"side\":\"HIDDEN\"},\"type\":\"ConnectorPlacement.EquallySpacedRectSide\",\"uuid\":\"f6309498-1e43-486f-b6b5-2c6570711f8e\"}]},\"type\":\"ConnectorPlacement.EquallySpacedConnector\",\"uuid\":\"f0ce492e-c9e1-4b35-98ef-84d77b696cfe\"}],\"packageUris\":[\"http://schema.mathworks.com/mf0/Connector/R2020b\"],\"version\":\"1.0\"}"
  HDL Data Descrambler : Subsystem
  QPSK Demodulator : Subsystem
  RRC Receive Filter : dsphdlfiltering2/Discrete FIR Filter  NumeratorSource=Property  Numerator=RRCCoef  NumeratorPrototype=[]  FilterStructure=Direct form systolic  SerializationOption=Minimum number of cycles between valid input samples  NumCycles=2  NumberOfMultipliers=2  SimulateUsing=Code generation  roundingMode=Floor  overflowMode=off  CoefficientsDataTypeStr=Inherit: Same word length as input  OutputDataTypeStr=Inherit: Same word length as input  ResetInputPort=off  HDLGlobalReset=off  CoeffMultiplier=Multiplier  UseMultForPow2Coeff=on  FrameInputSymmOptim=off
  dataOut : Outport
  ctrlOut : Outport  Port=2
  rxDiagBus : Outport  Port=3
  wires:
  Frequency and Time Synchronizer/6(normCoarseFreqEst) -> Bus Creator/2  "normCoarseFreqEst"
  HDL Data Descrambler/1(dataOut) -> dataOut/1
  HDL Data Descrambler/4(validOut) -> Bus Creator1/3  "validOut"
  QPSK Demodulator/1(dataOut) -> HDL Data Descrambler/1(dataIn)
  QPSK Demodulator/3(endOut) -> HDL Data Descrambler/3(endIn)
  QPSK Demodulator/4(validOut) -> HDL Data Descrambler/4(validIn)
  QPSK Demodulator/2(startOut) -> HDL Data Descrambler/2(startIn)
  Frequency and Time Synchronizer/1(dataOut) -> QPSK Demodulator/1(dataIn), Bus Creator/3  "QPSKConstellationPoints"
  Frequency and Time Synchronizer/4(validOut) -> QPSK Demodulator/4(validIn), Bus Creator/4  "QPSKConstellationValid"
  Frequency and Time Synchronizer/2(startOut) -> QPSK Demodulator/2(startIn)
  Frequency and Time Synchronizer/3(endOut) -> QPSK Demodulator/3(endIn)
  HDL Data Descrambler/3(endOut) -> Bus Creator1/2  "endOut"
  HDL Data Descrambler/2(startOut) -> Bus Creator1/1  "startOut"
  Bus Creator1/1 -> ctrlOut/1
  RRC Receive Filter/1 -> Frequency and Time Synchronizer/1(dataIn)
  RRC Receive Filter/2 -> Frequency and Time Synchronizer/2(validIn)
  Bus Creator/1 -> Delay/1
  Frequency and Time Synchronizer/5(nSynced) -> Bus Creator/1  "nSynced"
  Automatic Gain Control/2(validOut) -> RRC Receive Filter/2
  Automatic Gain Control/1(dataOut) -> RRC Receive Filter/1
  Delay/1 -> rxDiagBus/1
  rstCS/1 -> Frequency and Time Synchronizer/3(rstCS)
  ? -> FRFT Interference Cancellation/3(rstCS)
  FRFT Interference Cancellation/1(dataOut) -> ?
  ? -> FRFT Interference Cancellation/2(validIn)
  FRFT Interference Cancellation/2(validOut) -> ?
  ? -> FRFT Interference Cancellation/1(dataIn)
  dataIn/1 -> Automatic Gain Control/1(dataIn)
  validIn/1 -> Automatic Gain Control/2(validIn)

== system zynqRadioHWSWQPSKAD9361AD9364SL_orig/HDL_QPSK/QPSK Tx Channel QPSK Rx/QPSK Tx ==
  dataIn : Inport  OutDataTypeStr=boolean  PortDimensions=1
  validIn : Inport  Port=2  OutDataTypeStr=boolean  PortDimensions=1
  Bit Packetizer : Subsystem
  Bus Creator : BusCreator  Inputs=2
  HDL Data Scrambler : Subsystem
  QPSK Modulator : Subsystem
  RRC Transmit Filter : Subsystem
  dataReady : Outport
  dataOut : Outport  Port=2
  txDiagBus : Outport  Port=3
  validOut : Outport  Port=4
  wires:
  QPSK Modulator/1(dataOut) -> Bus Creator/1, RRC Transmit Filter/1(dataIn)  "QPSKConstellationPoints"
  QPSK Modulator/2(validOut) -> Bus Creator/2, RRC Transmit Filter/2(validIn)  "QPSKConstellationValid"
  Bit Packetizer/3(dataEnd) -> HDL Data Scrambler/3(endIn)
  Bit Packetizer/2(dataStart) -> HDL Data Scrambler/2(startIn)
  Bit Packetizer/1(bitsOut) -> HDL Data Scrambler/1(dataIn)
  Bit Packetizer/4(bitsValid) -> HDL Data Scrambler/4(validIn)
  HDL Data Scrambler/1(dataOut) -> QPSK Modulator/1(dataIn)
  HDL Data Scrambler/2(validOut) -> QPSK Modulator/2(validIn)
  Bit Packetizer/5(dataReady) -> dataReady/1
  RRC Transmit Filter/1(dataOut) -> dataOut/1
  RRC Transmit Filter/2(validOut) -> validOut/1
  Bus Creator/1 -> txDiagBus/1
  dataIn/1 -> Bit Packetizer/1(dataIn)
  validIn/1 -> Bit Packetizer/2(validIn)

== system zynqRadioHWSWQPSKAD9361AD9364SL_orig/HDL_QPSK/QPSK Tx Channel QPSK Rx/channel ==
  dataIn : Inport
  validIn : Inport  Port=2
  normalisedFreq : Inport  Port=3
  normalisedPhase : Inport  Port=4
  chirpEn : Inport  Port=5
  Add : Sum  OutDataTypeStr=Inherit: Same as first input
  Data Type Conversion : DataTypeConversion  OutDataTypeStr=fixdt(1,21,0)  ConvertRealWorld=Stored Integer (SI)  SaturateOnIntegerOverflow=off  RndMeth=Floor
  Data Type Conversion1 : DataTypeConversion  OutDataTypeStr=fixdt(1,21,0)  ConvertRealWorld=Stored Integer (SI)  SaturateOnIntegerOverflow=off  RndMeth=Floor
  Delay : Delay  DelayLength=6
  NCO HDL Optimized : dsphdlsigops2/NCO  PhaseIncrementSource=Input port  PhaseIncrement=100  PhaseOffsetSource=Input port  PhaseOffset=0  DitherSource=Property  NumDitherBits=11  SamplesPerFrame=1  LUTCompress=off  ResetAction=off  Waveform=Complex exponential  PhasePort=off  SimulateUsing=Code generation  AccumulatorWL=21  PhaseQuantization=on  NumQuantizerAccumulatorBits=14  OutputDataType=Binary point scaling  OutputWL=16  OutputFL=14
  NCO_DUT : Subsystem
  Product : Product  OutDataTypeStr=Inherit: Same as first input
  Real-Imag to Complex : RealImagToComplex
  Terminator{,1..3} (4 alike) : Terminator
  dataOut : Outport
  validOut : Outport  Port=2
  wires:
  validIn/1 -> NCO HDL Optimized/3
  dataIn/1 -> Delay/1
  NCO HDL Optimized/2 -> validOut/1
  normalisedFreq/1 -> Data Type Conversion/1
  Data Type Conversion/1 -> NCO HDL Optimized/1
  NCO HDL Optimized/1 -> Product/2
  Delay/1 -> Product/1
  Data Type Conversion1/1 -> NCO HDL Optimized/2
  normalisedPhase/1 -> Data Type Conversion1/1
  chirpEn/1 -> NCO_DUT/1(En_In)
  NCO_DUT/3(Address_Out) -> Terminator/1  "Address_Out"
  NCO_DUT/4(Address_Step_Out) -> Terminator1/1  "Address_Step_Out"
  NCO_DUT/5(Address_Step_Step_Out) -> Terminator2/1  "Address_Step_Step_Out"
  NCO_DUT/6(Reset_Out) -> Terminator3/1  "Reset_Out"
  Product/1 -> Add/1
  Add/1 -> dataOut/1
  NCO_DUT/1(NCO_Re_Out) -> Real-Imag to Complex/1  "NCO_Out"
  NCO_DUT/2(NCO_Im_Out) -> Real-Imag to Complex/2
  Real-Imag to Complex/1 -> Add/2

== system zynqRadioHWSWQPSKAD9361AD9364SL_orig/HDL_QPSK/Subsystem/BER ==
  userBitsValid : Inport
  resetcounter : Inport  Port=2
  reset : Inport  Port=3
  userBits : Inport  Port=4
  Capture Data Bits : Subsystem
  Compare To Constant : simulink/Logic and Bit Operations/Compare To Constant  relop===  const=0  OutDataTypeStr=boolean
  Data Type Conversion1 : DataTypeConversion  OutDataTypeStr=boolean  SaturateOnIntegerOverflow=off  RndMeth=Floor
  Delay : Delay  DelayLength=1
  Delay1 : Delay  DelayLength=1
  HDL Counter : hdlsllib/Sources/HDL Counter  CountType=Free running  CountInit=0  CountStep=1  CountMax=25  CountFromType=Initial value  CountFrom=0  CountResetPort=on  CountLoadPort=off  CountEnbPort=on  CountDirPort=off  CountHitOutputPort=off  CountDataType=Unsigned  CountWordLen=32  CountFracLen=0  CountSampTime=1
  HDL Counter1 : hdlsllib/Sources/HDL Counter  CountType=Free running  CountInit=0  CountStep=1  CountMax=25  CountFromType=Initial value  CountFrom=0  CountResetPort=on  CountLoadPort=off  CountEnbPort=on  CountDirPort=off  CountHitOutputPort=off  CountDataType=Unsigned  CountWordLen=32  CountFracLen=0  CountSampTime=1
  Logical Operator : Logic  AllPortsSameDT=off  OutDataTypeStr=boolean
  Logical Operator1 : Logic  Operator=OR  AllPortsSameDT=off  OutDataTypeStr=boolean
  Relational Operator : RelationalOperator  Operator=~=  OutDataTypeStr=boolean  InputSameDT=off
  Send Payload Data : Subsystem  TreatAsAtomicUnit=on
  bitCount : Outport  VectorParamsAs1DForOutWhenUnconnected=off
  bitErrors : Outport  Port=2  VectorParamsAs1DForOutWhenUnconnected=off
  wires:
  userBits/1 -> Delay1/1
  userBitsValid/1 -> Delay/1
  resetcounter/1 -> Send Payload Data/1(rst)
  Send Payload Data/1(dataIn) -> Data Type Conversion1/1
  Data Type Conversion1/1 -> Relational Operator/2
  Relational Operator/1 -> Logical Operator/2
  Logical Operator/1 -> HDL Counter/2
  HDL Counter1/1 -> Compare To Constant/1, bitCount/1
  HDL Counter/1 -> bitErrors/1
  Compare To Constant/1 -> Logical Operator1/1
  Logical Operator1/1 -> HDL Counter/1
  Delay/1 -> Send Payload Data/2(nxtBit), Logical Operator/1, HDL Counter1/2, Capture Data Bits/Enable
  Delay1/1 -> Relational Operator/1, Capture Data Bits/1(dataOut)
  reset/1 -> HDL Counter1/1, Logical Operator1/2

== system zynqRadioHWSWQPSKAD9361AD9364SL_orig/HDL_QPSK/Subsystem/Bits to Char ==
  data : Inport
  start : Inport  Port=2
  valid : Inport  Port=3
  Add : Sum  Inputs=++|  OutDataTypeStr=uint8  AccumDataTypeStr=uint8
  Bit Shift : hdlsllib/Logic and Bit Operations/Bit Shift  mode=Shift Left Logical  N=1
  Compare To Constant : simulink/Logic and Bit Operations/Compare To Constant  relop===  const=6  OutDataTypeStr=boolean
  Data Type Conversion1 : DataTypeConversion  OutDataTypeStr=fixdt(0,1,0)  SaturateOnIntegerOverflow=off  RndMeth=Floor
  Delay{,1..3} (4 alike) : Delay  DelayLength=1
  HDL Counter : hdlsllib/Sources/HDL Counter  CountType=Count limited  CountInit=0  CountStep=1  CountMax=6  CountFromType=Initial value  CountFrom=0  CountResetPort=on  CountLoadPort=off  CountEnbPort=on  CountDirPort=off  CountHitOutputPort=off  CountDataType=Unsigned  CountWordLen=3  CountFracLen=0  CountSampTime=1
  Logical Operator : Logic  AllPortsSameDT=off  OutDataTypeStr=boolean
  Unit Delay Enabled Resettable Synchronous : hdlsllib/Discrete/Unit Delay Enabled Resettable Synchronous  InitialCondition=0.0  SampleTime=-1
  charOut : Outport
  charValid : Outport  Port=2
  wires:
  data/1 -> Delay/1
  start/1 -> HDL Counter/1
  Unit Delay Enabled Resettable Synchronous/1 -> Bit Shift/1
  valid/1 -> Delay1/1
  Add/1 -> Delay3/1, Unit Delay Enabled Resettable Synchronous/1
  Bit Shift/1 -> Add/1
  Delay/1 -> Data Type Conversion1/1
  Data Type Conversion1/1 -> Add/2
  HDL Counter/1 -> Compare To Constant/1
  Logical Operator/1 -> Unit Delay Enabled Resettable Synchronous/3, Delay2/1
  Delay1/1 -> Unit Delay Enabled Resettable Synchronous/2, Logical Operator/2, HDL Counter/2
  Compare To Constant/1 -> Logical Operator/1
  Delay2/1 -> charValid/1
  Delay3/1 -> charOut/1

== system zynqRadioHWSWQPSKAD9361AD9364SL_orig/HDL_QPSK/QPSK Tx Channel QPSK Rx/QPSK Rx/Automatic Gain Control ==
  dataIn : Inport
  validIn : Inport  Port=2
  Data Type Duplicate : DataTypeDuplicate
  Data Type Conversion : DataTypeConversion  SaturateOnIntegerOverflow=off  RndMeth=Floor
  Delay{1..5} (5 alike) : Delay
  Error Detector : Subsystem
  Loop Filter : Subsystem
  Product : Product  OutDataTypeStr=Inherit: Same as first input
  dataOut : Outport
  validOut : Outport  Port=2
  wires:
  Data Type Conversion/1 -> Delay1/1, Data Type Duplicate/2
  Delay5/1 -> Delay3/1
  Delay3/1 -> validOut/1
  Delay4/1 -> Product/1
  Delay1/1 -> Product/2
  Loop Filter/1(gain) -> Data Type Conversion/1
  Error Detector/1(err) -> Loop Filter/1(err)
  validIn/1 -> Delay5/1
  Delay2/1 -> Error Detector/1(dataIn), dataOut/1
  dataIn/1 -> Delay4/1, Data Type Duplicate/1
  Product/1 -> Delay2/1

== system zynqRadioHWSWQPSKAD9361AD9364SL_orig/HDL_QPSK/QPSK Tx Channel QPSK Rx/QPSK Rx/FRFT Interference Cancellation ==
  dataIn : Inport
  validIn : Inport  Port=2
  rstCS : Inport  Port=3
  ChirpDDS : Subsystem
  FFT : dsphdlxfrm2/FFT  Architecture=Streaming Radix 2^2  FFTLengthSource=Property  FFTLength=1024  FFTLengthMax=1024  ComplexMultiplication=Use 4 multipliers and 2 adders  BitReversedOutput=on  BitReversedInput=off  Normalize=off  SimulateUsing=Code generation  RoundingMethod=Floor  ResetInputPort=on  StartOutputPort=on  EndOutputPort=on
  FIR FIlter : DiscreteFir  LoadFcn=dspblkCoreblockFVToolHelper(gcbh,'load');  ShowEnablePort=on
      settings: CopyFcn=dspblkCoreblockFVToolHelper(gcbh,'copy');  DeleteFcn=dspblkCoreblockFVToolHelper(gcbh,'close');  ModelCloseFcn=dspblkCoreblockFVToolHelper(gcbh,'close');  PreSaveFcn=dspblkCoreblockFVToolHelper(gcbh,'presave');  PostSaveFcn=dspblkCoreblockFVToolHelper(gcbh,'postsave');  CloseFcn=dspblkCoreblockFVToolHelper(gcbh,'close');  InputPortMap=u0,e7
  IFFT : dsphdlxfrm2/IFFT  Architecture=Streaming Radix 2^2  FFTLengthSource=Property  FFTLength=1024  FFTLengthMax=1024  ComplexMultiplication=Use 4 multipliers and 2 adders  BitReversedOutput=on  BitReversedInput=off  Normalize=on  SimulateUsing=Code generation  RoundingMethod=Floor  ResetInputPort=on  StartOutputPort=on  EndOutputPort=on
  Product : Product
  Switch : Switch  SaturateOnIntegerOverflow=off  InputSameDT=off
  dataOut : Outport
  validOut : Outport  Port=2
